simulink model "Lab1_REDO_before_PID"  (R2014b)
settings: Solver=ode45  StartTime=0.0  StopTime=10.0  RelTol=1e-3
undefined symbols (not defined in the file): b, g, I, l, L, M, m
settings Model: Creator=nrjbasu  LastModifiedBy=nrjbasu

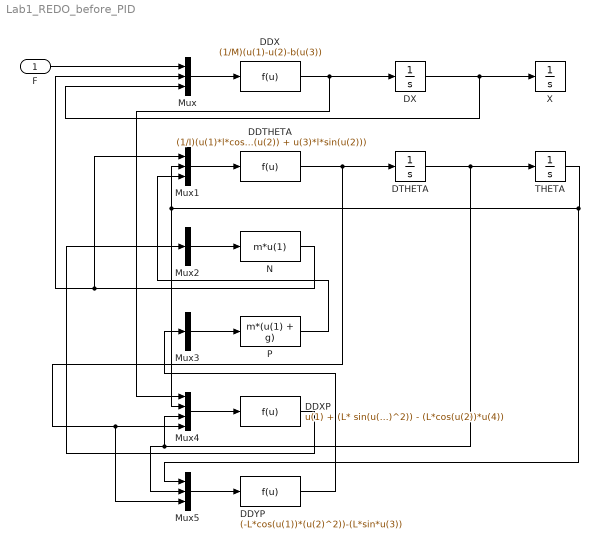
== system Lab1_REDO_before_PID ==
  F : Inport
  DDTHETA : Fcn  Expr=(1/I)(u(1)*l*cos(u(2)) + u(3)*l*sin(u(2)))
  DDX : Fcn  Expr=(1/M)(u(1)-u(2)-b(u(3))
  DDXP : Fcn  Expr=u(1) + (L* sin(u(2))*(u(3)^2)) - (L*cos(u(2))*u(4))
  DDYP : Fcn  Expr=(-L*cos(u(1))*(u(2)^2))-(L*sin*u(3))
  DTHETA : Integrator
  DX : Integrator
  Mux : Mux  Inputs=3
  Mux1 : Mux  Inputs=3
  Mux2 : Mux  Inputs=1
  Mux3 : Mux  Inputs=1
  Mux4 : Mux
  Mux5 : Mux  Inputs=3
  N : Fcn  Expr=m*u(1)
  P : Fcn  Expr=m*(u(1) + g)
  THETA : Integrator
  X : Integrator
  wires:
  Mux/1 -> DDX/1
  Mux1/1 -> DDTHETA/1
  Mux2/1 -> N/1
  Mux3/1 -> P/1
  Mux4/1 -> DDXP/1
  Mux5/1 -> DDYP/1
  DDX/1 -> Mux4/1, DX/1
  DX/1 -> Mux/3, X/1
  DDTHETA/1 -> Mux5/3, Mux4/4, DTHETA/1
  DTHETA/1 -> Mux5/2, Mux4/3, THETA/1
  F/1 -> Mux/1
  N/1 -> Mux1/1, Mux/2
  THETA/1 -> Mux5/1, Mux4/2, Mux1/2
  P/1 -> Mux1/3
  DDXP/1 -> Mux2/1
  DDYP/1 -> Mux3/1
